simulink model "Kalman_Filter_Simulink_Example_EKF"  (R2018a)
settings: Solver=FixedStepAuto  StartTime=0.0  StopTime=30  FixedStep=0.001  RelTol=1e-3
values from neighbouring files (symbols this model uses):
  g = 9.81    [Kalman_Filter_Simulink_Example_params_EKF.m]
  l = 0.5    [Kalman_Filter_Simulink_Example_params_EKF.m]
  P0 = [10 0; 0 10]    [Kalman_Filter_Simulink_Example_params_EKF.m]
  Q = 1e-4    (= 0.0001)    [Kalman_Filter_Simulink_Example_params_EKF.m]
  Q0 = 2e-4    (= 0.0002)    [Kalman_Filter_Simulink_Example_params_EKF.m]
  R = 1e-3    (= 0.001)    [Kalman_Filter_Simulink_Example_params_EKF.m]
  R0 = 2e-3    (= 0.002)    [Kalman_Filter_Simulink_Example_params_EKF.m]
  theta0 = pi/4    (= 0.785398163397)    [Kalman_Filter_Simulink_Example_params_EKF.m]
  Ts = 0.01    [Kalman_Filter_Simulink_Example_params_EKF.m]
libraries: simulink x3, sharedTrackingLibrary x1, Meldas_Library x1
settings Model: Creator=mulusoy  LastModifiedBy=hussein
settings OptimizationCC: DefaultParameterBehavior=Inlined  PassReuseOutputArgsAs=Individual arguments
settings DebuggingCC: ParameterTunabilityLossMsg=error
settings SFSimCC: MATLABDynamicMemAlloc=off
settings RTWCC: SystemTargetFile=ert.tlc  TemplateMakefile=ert_default_tmf  GenerateReport=on  IncludeHyperlinkInReport=on  LaunchReport=on  GenerateTraceInfo=on  GenerateTraceReport=on  GenerateTraceReportSl=on  GenerateTraceReportSf=on  GenerateTraceReportEml=on  CheckMdlBeforeBuild=Warning
settings CodeAppCC: GenerateComments=off  IgnoreCustomStorageClasses=off  SimulinkBlockComments=off
settings ERTTargetCC: TargetLangStandard=C99 (ISO)  GenerateSampleERTMain=on  InlinedParameterPlacement=NonHierarchical  ERTCustomFileTemplate=example_file_process.tlc
settings SimscapeCC: SimscapeNormalizeSystem=off

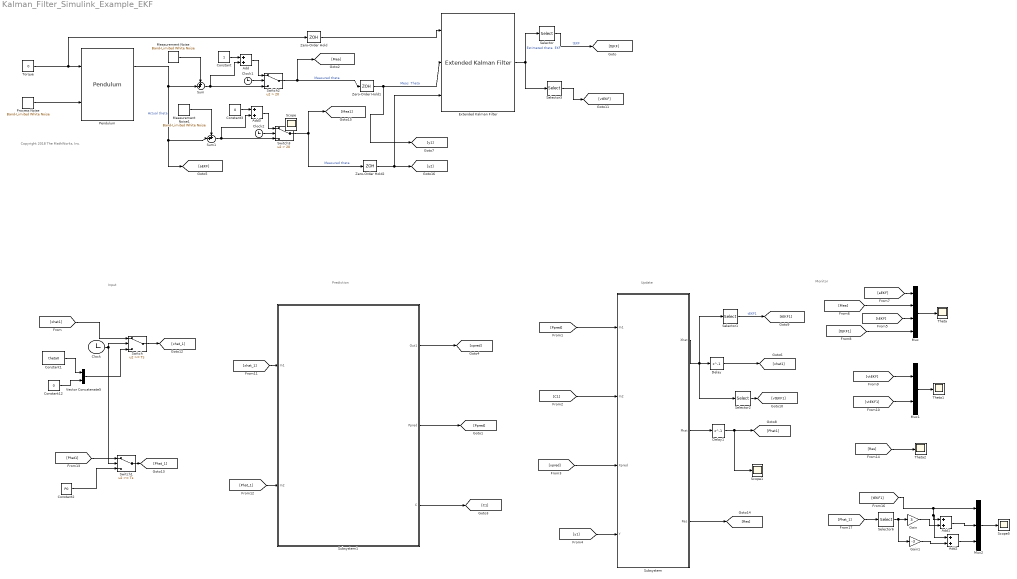
== system Kalman_Filter_Simulink_Example_EKF ==
  note: Monitor
  note: Input
  note: Update
  note: Prediction
  note: Copyright 2018 The MathWorks, Inc.
  Add{,1..3} (4 alike) : Sum
  Clock : Clock
      settings: Decimation=1000
  Clock1 : Clock
  Clock2 : Clock
  Constant : Constant
  Constant1 : Constant  Value=theta0
  Constant12 : Constant  Value=0
  Constant2 : Constant  Value=P0
  Constant3 : Constant  Value=0
  Delay : Delay  DelayLength=1  SampleTime=Ts
  Delay1 : Delay  DelayLength=1  SampleTime=Ts
  Extended Kalman Filter : sharedTrackingLibrary/Extended Kalman Filter  StateTransitionFcn=myStateTransitionFcn  HasStateTransitionJacobianFcn=off  HasAdditiveProcessNoise=Additive  ProcessNoise=diag([0,Q0])  HasTimeVaryingProcessNoise=off  HasStateTransitionFcnExtraArgument=1  InitialState=[pi/2 0]  InitialStateCovariance=1e-6  MeasurementFcn1=myMeasurementFcn  HasMeasurementJacobianFcn1=off  HasMeasurementEnablePort1=off  HasAdditiveMeasurementNoise1=Additive  MeasurementNoise1=R0  HasTimeVaryingMeasurementNoise1=off  HasMeasurementFcnExtraArgument1=0  MeasurementFcn2=myMeasurementFcn  HasMeasurementJacobianFcn2=off  HasMeasurementEnablePort2=off  HasAdditiveMeasurementNoise2=Additive  MeasurementNoise2=R0  HasTimeVaryingMeasurementNoise2=off  HasMeasurementFcnExtraArgument2=0  MeasurementFcn3=myMeasurementFcn  HasMeasurementJacobianFcn3=off  HasMeasurementEnablePort3=off  HasAdditiveMeasurementNoise3=Additive  MeasurementNoise3=1  HasTimeVaryingMeasurementNoise3=off  HasMeasurementFcnExtraArgument3=0  MeasurementFcn4=myMeasurementFcn  HasMeasurementJacobianFcn4=off  HasMeasurementEnablePort4=off  HasAdditiveMeasurementNoise4=Additive  MeasurementNoise4=1  HasTimeVaryingMeasurementNoise4=off  HasMeasurementFcnExtraArgument4=0  MeasurementFcn5=myMeasurementFcn  HasMeasurementJacobianFcn5=off  HasMeasurementEnablePort5=off  HasAdditiveMeasurementNoise5=Additive  MeasurementNoise5=1  HasTimeVaryingMeasurementNoise5=off  HasMeasurementFcnExtraArgument5=0  EnableMultirate=off  StateTransitionFcnSampleTime=1  MeasurementFcn1SampleTime=1  MeasurementFcn2SampleTime=1  MeasurementFcn3SampleTime=1  MeasurementFcn4SampleTime=1  MeasurementFcn5SampleTime=1  UseCurrentEstimator=on  OutputStateCovariance=off  DataType=double  SampleTime=Ts  NumberOfMeasurements=2
      settings: SourceProductName=Control System Toolbox  SourceProductBaseCode=CT
  Gain : Gain  Gain=3
  Gain1 : Gain  Gain=-3
  Measurement Noise : simulink/Sources/Band-Limited White Noise  Cov=R*Ts  Ts=Ts  seed=[12347]
  Measurement Noise1 : simulink/Sources/Band-Limited White Noise  Cov=R*Ts  Ts=Ts  seed=[12347]
  Mux : Mux
  Mux1 : Mux  Inputs=2
  Mux2 : Mux  Inputs=3
  Pendulum : Meldas_Library/Pendulum  theta_0=pi/2  theta_dot_0=0
  Process Noise : simulink/Sources/Band-Limited White Noise  Cov=Q*Ts  Ts=Ts  seed=[23341]
  Scope1 : Scope
  Scope5 : Scope
  Selector : Selector  InputPortWidth=2  IndexOptions=Index vector (dialog)  Indices=1  OutputSizes=1
  Selector1 : Selector  InputPortWidth=2  IndexOptions=Index vector (dialog)  Indices=1  OutputSizes=1
  Selector2 : Selector  InputPortWidth=2  IndexOptions=Index vector (dialog)  Indices=2  OutputSizes=1
  Selector3 : Selector  InputPortWidth=2  IndexOptions=Index vector (dialog)  Indices=2  OutputSizes=1
  Selector6 : Selector  NumberOfDimensions=2  InputPortWidth=3  IndexOptions=Index vector (dialog),Index vector (dialog)  Indices=1,1  OutputSizes=1,1
  Subsystem : Subsystem
  Subsystem1 : Subsystem
  Sum : Sum  Inputs=++|
  Sum1 : Sum  Inputs=++|
  Switch : Switch  Threshold=Ts
  Switch1 : Switch  Threshold=Ts
  Switch2 : Switch  Criteria=u2 > Threshold  Threshold=20
  Switch3 : Switch  Criteria=u2 > Threshold  Threshold=20
  Theta : Scope
  Theta1 : Scope
  Theta2 : Scope
  Torque : Constant  Value=0
  Vector Concatenate5 : Concatenate
  Zero-Order Hold : ZeroOrderHold  SampleTime=Ts
  Zero-Order Hold1 : ZeroOrderHold  SampleTime=Ts
  Zero-Order Hold2 : ZeroOrderHold  SampleTime=Ts
  Scope : Scope
  wires:
  Sum/1 -> Add/2, Switch2/3
  Torque/1 -> Pendulum/1, Zero-Order Hold/1
  Zero-Order Hold/1 -> Extended Kalman Filter/1
  Zero-Order Hold1/1 -> [y1], Extended Kalman Filter/2  "Meas  Theta"
  Extended Kalman Filter/1 -> Selector/1, Selector3/1  "Estimated theta  EKF"
  Clock/1 -> Switch1/2, Switch/2
  Constant1/1 -> Vector Concatenate5/1
  Constant2/1 -> Switch1/3
  Constant12/1 -> Vector Concatenate5/2
  Vector Concatenate5/1 -> Switch/3
  Measurement Noise/1 -> Sum/1
  Process Noise/1 -> Pendulum/2
  [xhat1] -> Switch/1
  [Phat1] -> Switch1/1
  [Ppred] -> Subsystem/1(In1)
  [C1] -> Subsystem/2(In2)
  [xpred] -> Subsystem/3(Xpred)
  Subsystem/2("Phat ") -> Delay1/1
  [y1] -> Subsystem/4("Y ")
  Subsystem1/1(Out1) -> [xpred]
  Subsystem1/2(Ppred) -> [Ppred]
  Subsystem1/3("C ") -> [C1]
  Delay1/1 -> Scope1/1, [Phat1]
  Constant/1 -> Add/1
  Add/1 -> Switch2/1
  Switch2/1 -> [Mea], Zero-Order Hold1/1  "Measured theta"
  Clock1/1 -> Switch2/2
  Delay/1 -> [xhat1]
  Selector/1 -> [tEKF]  "tEKF"
  Selector1/1 -> [tEKF1]  "tEKF1"
  Selector2/1 -> [vtEKF1]
  Selector3/1 -> [vtEKF]
  [xhat_1] -> Subsystem1/1(In1)
  Switch/1 -> [xhat_1]
  [Phat_1] -> Subsystem1/2(In2)
  Switch1/1 -> [Phat_1]
  [tEKF] -> Mux/3
  [aEKF] -> Mux/1
  [Mea] -> Mux/2
  [vtEKF] -> Mux1/1
  Mux1/1 -> Theta1/1
  [tEKF1] -> Mux/4
  [vtEKF1] -> Mux1/2
  Mux/1 -> Theta/1
  Subsystem/3(Res) -> [Res]
  [Res] -> Theta2/1
  Mux2/1 -> Scope5/1
  Gain1/1 -> Add2/2
  Gain/1 -> Add1/2
  [tEKF1] -> Add2/1, Add1/1, Mux2/1
  Add2/1 -> Mux2/3
  Selector6/1 -> Gain1/1, Gain/1
  Add1/1 -> Mux2/2
  [Phat_1] -> Selector6/1
  Subsystem/1(Xhat) -> Selector2/1, Selector1/1, Delay/1
  Clock2/1 -> Switch3/2
  Pendulum/1 -> Sum1/2, [aEKF], Sum/2  "Actual theta"
  Constant3/1 -> Add3/1
  Sum1/1 -> Add3/2, Switch3/3
  Measurement Noise1/1 -> Sum1/1
  Add3/1 -> Switch3/1
  Switch3/1 -> Zero-Order Hold2/1, [Mea1]  "Measured theta"
  Zero-Order Hold2/1 -> Extended Kalman Filter/3, [y2]

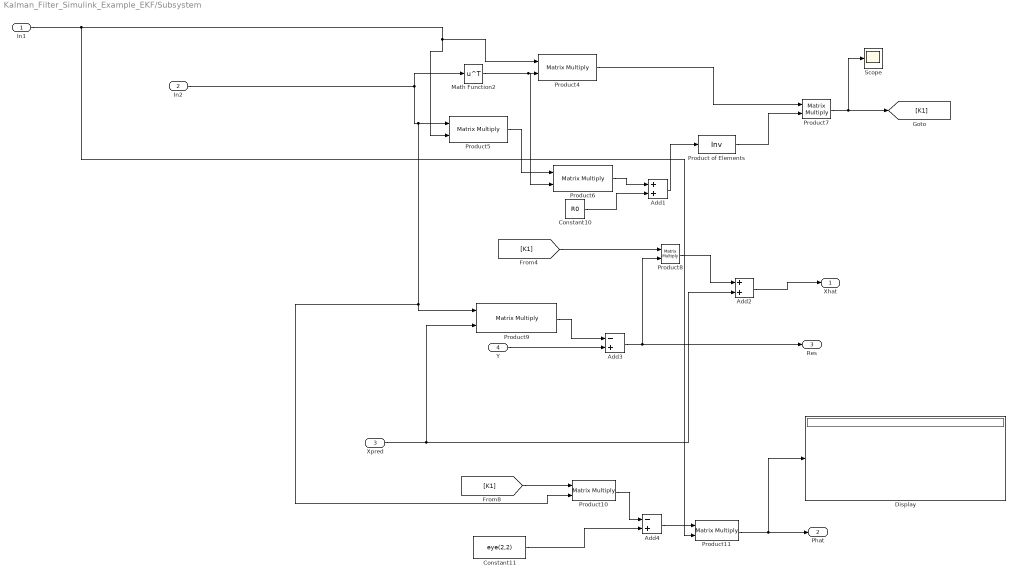
== system Kalman_Filter_Simulink_Example_EKF/Subsystem ==
  In1 : Inport
  In2 : Inport  Port=2
  Xpred : Inport  Port=3
  "Y " : Inport  Port=4
  Add1 : Sum
  Add2 : Sum
  Add3 : Sum  Inputs=-+
  Add4 : Sum  Inputs=-+
  Constant10 : Constant  Value=R0
  Constant11 : Constant  Value=eye(2,2)
  Display : Display
  Math Function2 : Math  Operator=transpose  SaturateOnIntegerOverflow=on
  Product of Elements : Product  Inputs=/  Multiplication=Matrix(*)
  Product{4..11} (8 alike) : Product  Multiplication=Matrix(*)
  Scope : Scope
  Xhat : Outport  PortDimensions=[2,1]
  "Phat " : Outport  Port=2
  Res : Outport  Port=3  PortDimensions=1
  wires:
  Product5/1 -> Product6/1
  Math Function2/1 -> Product6/2, Product4/2
  Product4/1 -> Product7/1
  Xpred/1 -> Product9/2, Add2/2
  In2/1 -> Math Function2/1, Product10/2, Product9/1, Product5/1
  Add1/1 -> Product of Elements/1
  [K1] -> Product8/1
  Product9/1 -> Add3/1
  Add4/1 -> Product11/1
  Product10/1 -> Add4/1
  Product8/1 -> Add2/1
  In1/1 -> Product11/2, Product4/1, Product5/2
  [K1] -> Product10/1
  "Y "/1 -> Add3/2
  Constant11/1 -> Add4/2
  Add3/1 -> Res/1, Product8/2
  Product6/1 -> Add1/1
  Add2/1 -> Xhat/1
  Product11/1 -> Display/1, "Phat "/1
  Product7/1 -> Scope/1, [K1]
  Constant10/1 -> Add1/2
  Product of Elements/1 -> Product7/2

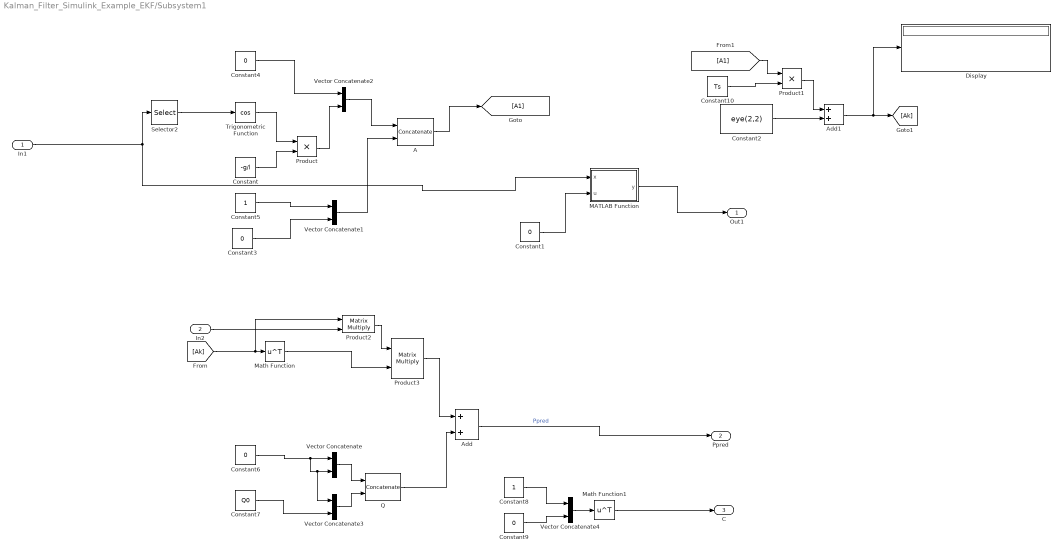
== system Kalman_Filter_Simulink_Example_EKF/Subsystem1 ==
  In1 : Inport
  In2 : Inport  Port=2
  A : Concatenate  Mode=Multidimensional array  ConcatenateDimension=2
  Add : Sum
  Add1 : Sum
  Constant : Constant  Value=-g/l
  Constant{1,3..4,6,9} (5 alike) : Constant  Value=0
  Constant10 : Constant  Value=Ts
  Constant2 : Constant  Value=eye(2,2)
  Constant5 : Constant
  Constant7 : Constant  Value=Q0
  Constant8 : Constant
  Display : Display
  MATLAB Function : MATLAB Function  TreatAsAtomicUnit=on
  Math Function : Math  Operator=transpose  SaturateOnIntegerOverflow=on
  Math Function1 : Math  Operator=transpose  SaturateOnIntegerOverflow=on
  Product : Product
  Product1 : Product
  Product2 : Product  Multiplication=Matrix(*)
  Product3 : Product  Multiplication=Matrix(*)
  Q : Concatenate  Mode=Multidimensional array  ConcatenateDimension=2
  Selector2 : Selector  InputPortWidth=2  IndexOptions=Index vector (dialog)  Indices=1  OutputSizes=1
  Trigonometric Function : Trigonometry  Operator=cos
  Vector Concatenate{,1..4} (5 alike) : Concatenate
  Out1 : Outport
  Ppred : Outport  Port=2
  "C " : Outport  Port=3
  wires:
  Constant3/1 -> Vector Concatenate1/2
  Product3/1 -> Add/1
  Selector2/1 -> Trigonometric Function/1
  Vector Concatenate2/1 -> A/1
  Constant/1 -> Product/2
  Constant6/1 -> Vector Concatenate3/1, Vector Concatenate/2, Vector Concatenate/1
  Trigonometric Function/1 -> Product/1
  Vector Concatenate1/1 -> A/2
  Math Function/1 -> Product3/2
  In2/1 -> Product2/2
  Product2/1 -> Product3/1
  Product/1 -> Vector Concatenate2/2
  Vector Concatenate4/1 -> Math Function1/1
  [Ak] -> Product2/1, Math Function/1
  Q/1 -> Add/2
  Constant9/1 -> Vector Concatenate4/2
  Add/1 -> Ppred/1  "Ppred"
  Constant5/1 -> Vector Concatenate1/1
  Constant7/1 -> Vector Concatenate3/2
  Constant4/1 -> Vector Concatenate2/1
  Vector Concatenate3/1 -> Q/2
  Constant8/1 -> Vector Concatenate4/1
  A/1 -> [A1]
  Vector Concatenate/1 -> Q/1
  Math Function1/1 -> "C "/1
  In1/1 -> Selector2/1, MATLAB Function/1(x)
  MATLAB Function/1(y) -> Out1/1
  Constant1/1 -> MATLAB Function/2(u)
  Constant10/1 -> Product1/2
  [A1] -> Product1/1
  Add1/1 -> Display/1, [Ak]
  Product1/1 -> Add1/1
  Constant2/1 -> Add1/2

== matlab function Kalman_Filter_Simulink_Example_EKF/Subsystem1/MATLAB Function ==
  data: x input; u input; y output
function y =Trans(x,u)

dt = 0.01;

y= x + [x(2); -9.81/0.5*sin(x(1))+u]*dt;
end
